simulink model "automata_learning"  (R2022a)
settings: Solver=FixedStepAuto  StartTime=0.0  StopTime=10.0  FixedStep=0.01  RelTol=1e-3
settings Model: Creator=diego  LastModifiedBy=diego

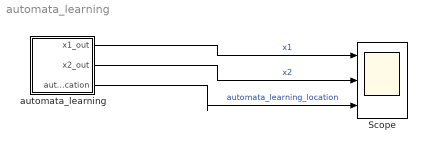
== system automata_learning ==
  Scope : Scope  NumInputPorts=3
  automata_learning : Stateflow chart  TreatAsAtomicUnit=on
  wires:
  automata_learning/1(x1_out) -> Scope/1  "x1"
  automata_learning/2(x2_out) -> Scope/2  "x2"
  automata_learning/3(automata_learning_location) -> Scope/3  "automata_learning_location"

== stateflow chart automata_learning/automata_learning ==
  settings: updateMethod=CONTINUOUS
  state loc1
    du:
    x1_dot = 0.0000009001406845437349 - 0.9999960669356369 * x2 - 0.0000007631377191633093 * x1;
    x2_dot = 0.8776739059467218 * x1 + 0.012313356278895071 * x2 + 0.5176177851772081;
    x1_out=x1;
    x2_out=x2;
    automata_learning_location =1;
  state loc2
    du:
    x1_dot = -0.000008342971326819049 * x1 - 0.9999939545105008 * x2 - 0.000011790638267755726;
    x2_dot = 6.093528869838337 * x1 + 0.004641196259910885 * x2 + 5.569810735149076;
    x1_out=x1;
    x2_out=x2;
    automata_learning_location =2;
  loc1 -> loc2 : [0.3288 * x1 - 0.333 * x2 + 1.0 < 0.0]
  (default) -> loc1 : {x1 = 1.0;
      | x2 = -1.0;}
  loc2 -> loc1 : [0.499 * x2 - 0.0006802 * x1 + 1.0 < 0.0]
  data: x1_out output; x1 local; x2_out output; x2 local; automata_learning_location output
  data x1 settings: updateMethod=SF_CONTINUOUS_TIME_DATA
  data x2 settings: updateMethod=SF_CONTINUOUS_TIME_DATA
